simulink model "FIRST_SIMULATION"  (R2016a)
settings: Solver=ode45  SolverMode=SingleTasking  StartTime=0.0  StopTime=5/60  RelTol=1e-3
libraries: powerlib x63, powerlib_meascontrol x44
settings Model: Creator=hiago  LastModifiedBy=hiago
settings DebuggingCC: SFUnexpectedBacktrackingDiag=error  SFNoUnconditionalDefaultTransitionDiag=error
settings SFSimCC: SimUseLocalCustomCode=on
settings RTWCC: RTWUseLocalCustomCode=on
settings GRTTargetCC: TargetLangStandard=C99 (ISO)  GeneratePreprocessorConditionals=Use local settings
settings ConfigComp: CovMetricSettings=dwe  CovHtmlReporting=off  CovSaveCumulativeToWorkspaceVar=off  CovSaveSingleToWorkspaceVar=off  CovExternalEMLEnable=on

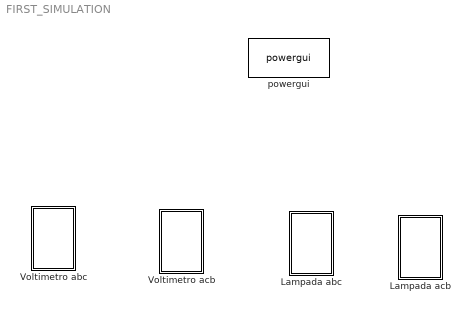
== system FIRST_SIMULATION ==
  Lampada abc : Subsystem
  Lampada acb : Subsystem
  Voltimetro abc : Subsystem
  Voltimetro acb : Subsystem
  powergui : powerlib/powergui  Priority=1  SimulationMode=Discrete  SampleTime=50e-6  frequency=60  Iterations=50  frequencyindice=60  Pbase=100e6  ErrMax=1e-4  UnitsV=kV  UnitsW=MW  buscounter=0  FunctionMessages=off  echomessages=off  EnableUseOfTLC=off  CurrentSourceSwitches=off  DisableSnubberDevices=off  DisableRonSwitches=off  DisableVfSwitches=off  DisplayEquations=off  SolverType=Tustin/Backward Euler (TBE)  Interpol=off  ExternalGateDelay=off  methode=off  Ts=100  x0status=blocks  SPID=on  SwTol=0  HookPort=off  RestoreLinks=warning  ResistiveCurrentMeasurement=off  Frange=[0:2:500]  Ylog=off  Xlog=on  ShowGrid=off  save=off  variable=ZData  structure=0  ZoomFFT=off  StartTime=0.0  cycles=1  DisplayStyle=1  fundamental=60  FreqAxis=off  MaxFrequency=1000  frequencyindicesteady=1  RmsSteady=1  display=off

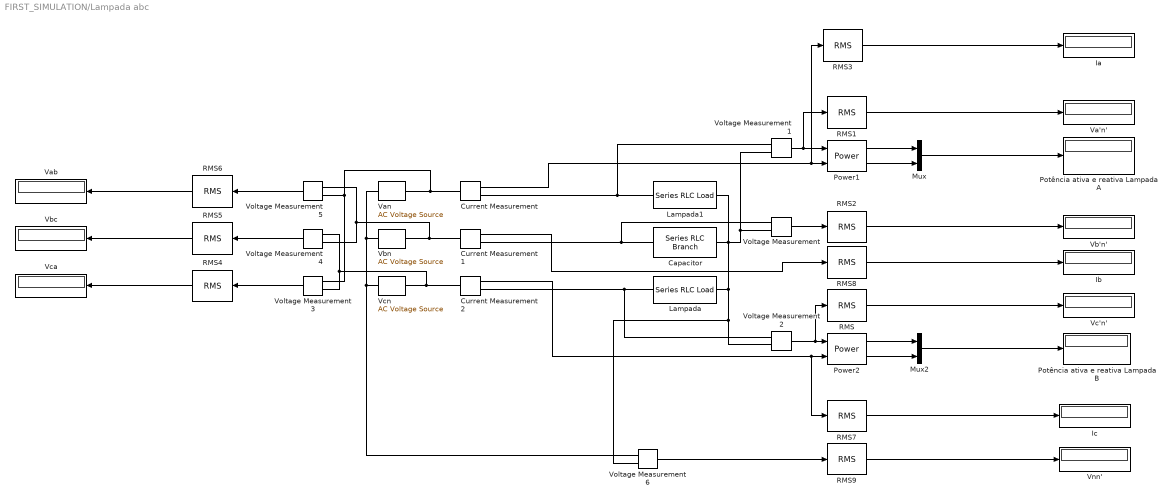
== system FIRST_SIMULATION/Lampada abc ==
  Capacitor : powerlib/Elements/Series RLC Branch  LConnTagsString=__new0  RConnTagsString=__new0  BranchType=RC  Resistance=0.0000001  Inductance=1e-3  SetiL0=off  InitialCurrent=0  Capacitance=25e-6  Setx0=off  InitialVoltage=0  Measurements=None
  Current Measurement : powerlib/Measurements/Current Measurement  PhasorSimulation=off  OutputType=Complex  PSBequivalent=0
  Current Measurement1 : powerlib/Measurements/Current Measurement  PhasorSimulation=off  OutputType=Complex  PSBequivalent=0
  Current Measurement2 : powerlib/Measurements/Current Measurement  PhasorSimulation=off  OutputType=Complex  PSBequivalent=0
  Ia : Display
  Ib : Display
  Ic : Display
  Lampada : powerlib/Elements/Series RLC Load  LConnTagsString=a  RConnTagsString=__new0  NominalVoltage=220  NominalFrequency=60  ActivePower=150  InductivePower=0  CapacitivePower=0  Setx0=off  InitialVoltage=0  SetiL0=off  InitialCurrent=0  Measurements=None  LoadType=constant Z
  Lampada1 : powerlib/Elements/Series RLC Load  LConnTagsString=a  RConnTagsString=__new0  NominalVoltage=220  NominalFrequency=60  ActivePower=150  InductivePower=0  CapacitivePower=0  Setx0=off  InitialVoltage=0  SetiL0=off  InitialCurrent=0  Measurements=None  LoadType=constant Z
  Mux : Mux  Inputs=2
  Mux2 : Mux  Inputs=2
  Potência ativa e reativa Lampada A : Display
  Potência ativa e reativa Lampada B : Display
  Power1 : powerlib_meascontrol/Measurements/Power  Freq=60  Vinit=[1, 0]  Iinit=[1, 0]  Ts=5e-5
  Power2 : powerlib_meascontrol/Measurements/Power  Freq=60  Vinit=[1, 0]  Iinit=[1, 0]  Ts=5e-5
  RMS{,1..9} (10 alike) : powerlib_meascontrol/Measurements/RMS  TrueRMS=on  Freq=60  RMSInit=120  Ts=5e-5
  Va'n' : Display
  Vab : Display
  Van : powerlib/Electrical Sources/AC Voltage Source  Amplitude=127*sqrt(2)  Phase=0  Frequency=60  SampleTime=5e-5  Measurements=None  BusType=swing  Pref=10e3  Qref=0  Qmin=-inf  Qmax=+inf
  Vb'n' : Display
  Vbc : Display
  Vbn : powerlib/Electrical Sources/AC Voltage Source  Amplitude=127*sqrt(2)  Phase=-120  Frequency=60  SampleTime=5e-5  Measurements=None  BusType=swing  Pref=10e3  Qref=0  Qmin=-inf  Qmax=+inf
  Vc'n' : Display
  Vca : Display
  Vcn : powerlib/Electrical Sources/AC Voltage Source  Amplitude=127*sqrt(2)  Phase=120  Frequency=60  SampleTime=5e-5  Measurements=None  BusType=swing  Pref=10e3  Qref=0  Qmin=-inf  Qmax=+inf
  Vnn' : Display
  Voltage Measurement{,1..6} (7 alike) : powerlib/Measurements/Voltage Measurement  PhasorSimulation=off  OutputType=Complex  PSBequivalent=0
  wires:
  Voltage Measurement2/1 -> RMS/1, Power2/1
  Current Measurement2/1 -> RMS7/1, Power2/2
  Voltage Measurement1/1 -> RMS1/1, Power1/1
  Current Measurement/1 -> RMS3/1, Power1/2
  Voltage Measurement/1 -> RMS2/1
  RMS1/1 -> Va'n'/1
  RMS2/1 -> Vb'n'/1
  RMS/1 -> Vc'n'/1
  Power1/1 -> Mux/1
  Power1/2 -> Mux/2
  Power2/1 -> Mux2/1
  Power2/2 -> Mux2/2
  Mux2/1 -> Potência ativa e reativa Lampada B/1
  Mux/1 -> Potência ativa e reativa Lampada A/1
  RMS6/1 -> Vab/1
  RMS5/1 -> Vbc/1
  Voltage Measurement3/1 -> RMS4/1
  Voltage Measurement5/1 -> RMS6/1
  Voltage Measurement4/1 -> RMS5/1
  RMS4/1 -> Vca/1
  RMS3/1 -> Ia/1
  RMS7/1 -> Ic/1
  RMS8/1 -> Ib/1
  Current Measurement1/1 -> RMS8/1
  RMS9/1 -> Vnn'/1
  Voltage Measurement6/1 -> RMS9/1
  connections:
  Lampada/LConn1 -- Current Measurement2/RConn1 -- Voltage Measurement2/LConn1
  Lampada1/RConn1 -- Voltage Measurement6/LConn2 -- Voltage Measurement2/LConn2 -- Lampada/RConn1 -- Voltage Measurement/LConn2 -- Voltage Measurement1/LConn2 -- Capacitor/RConn1
  Vcn/LConn1 -- Voltage Measurement6/LConn1 -- Van/LConn1 -- Vbn/LConn1
  Current Measurement/LConn1 -- Voltage Measurement3/LConn2 -- Voltage Measurement5/LConn1 -- Van/RConn1
  Current Measurement/RConn1 -- Voltage Measurement1/LConn1 -- Lampada1/LConn1
  Current Measurement1/LConn1 -- Voltage Measurement4/LConn1 -- Voltage Measurement5/LConn2 -- Vbn/RConn1
  Current Measurement1/RConn1 -- Voltage Measurement/LConn1 -- Capacitor/LConn1
  Current Measurement2/LConn1 -- Voltage Measurement3/LConn1 -- Voltage Measurement4/LConn2 -- Vcn/RConn1

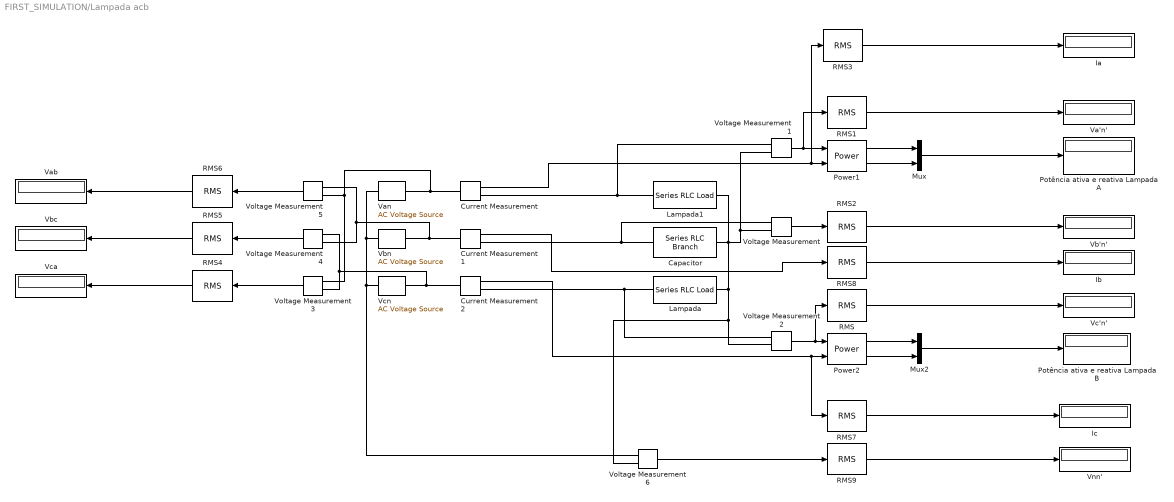
== system FIRST_SIMULATION/Lampada acb ==
  Capacitor : powerlib/Elements/Series RLC Branch  LConnTagsString=__new0  RConnTagsString=__new0  BranchType=RC  Resistance=0.0000001  Inductance=1e-3  SetiL0=off  InitialCurrent=0  Capacitance=25e-6  Setx0=off  InitialVoltage=0  Measurements=None
  Current Measurement : powerlib/Measurements/Current Measurement  PhasorSimulation=off  OutputType=Complex  PSBequivalent=0
  Current Measurement1 : powerlib/Measurements/Current Measurement  PhasorSimulation=off  OutputType=Complex  PSBequivalent=0
  Current Measurement2 : powerlib/Measurements/Current Measurement  PhasorSimulation=off  OutputType=Complex  PSBequivalent=0
  Ia : Display
  Ib : Display
  Ic : Display
  Lampada : powerlib/Elements/Series RLC Load  LConnTagsString=a  RConnTagsString=__new0  NominalVoltage=220  NominalFrequency=60  ActivePower=150  InductivePower=0  CapacitivePower=0  Setx0=off  InitialVoltage=0  SetiL0=off  InitialCurrent=0  Measurements=None  LoadType=constant Z
  Lampada1 : powerlib/Elements/Series RLC Load  LConnTagsString=a  RConnTagsString=__new0  NominalVoltage=220  NominalFrequency=60  ActivePower=150  InductivePower=0  CapacitivePower=0  Setx0=off  InitialVoltage=0  SetiL0=off  InitialCurrent=0  Measurements=None  LoadType=constant Z
  Mux : Mux  Inputs=2
  Mux2 : Mux  Inputs=2
  Potência ativa e reativa Lampada A : Display
  Potência ativa e reativa Lampada B : Display
  Power1 : powerlib_meascontrol/Measurements/Power  Freq=60  Vinit=[1, 0]  Iinit=[1, 0]  Ts=5e-5
  Power2 : powerlib_meascontrol/Measurements/Power  Freq=60  Vinit=[1, 0]  Iinit=[1, 0]  Ts=5e-5
  RMS{,1..9} (10 alike) : powerlib_meascontrol/Measurements/RMS  TrueRMS=on  Freq=60  RMSInit=120  Ts=5e-5
  Va'n' : Display
  Vab : Display
  Van : powerlib/Electrical Sources/AC Voltage Source  Amplitude=127*sqrt(2)  Phase=0  Frequency=60  SampleTime=5e-5  Measurements=None  BusType=swing  Pref=10e3  Qref=0  Qmin=-inf  Qmax=+inf
  Vb'n' : Display
  Vbc : Display
  Vbn : powerlib/Electrical Sources/AC Voltage Source  Amplitude=127*sqrt(2)  Phase=120  Frequency=60  SampleTime=5e-5  Measurements=None  BusType=swing  Pref=10e3  Qref=0  Qmin=-inf  Qmax=+inf
  Vc'n' : Display
  Vca : Display
  Vcn : powerlib/Electrical Sources/AC Voltage Source  Amplitude=127*sqrt(2)  Phase=-120  Frequency=60  SampleTime=5e-5  Measurements=None  BusType=swing  Pref=10e3  Qref=0  Qmin=-inf  Qmax=+inf
  Vnn' : Display
  Voltage Measurement{,1..6} (7 alike) : powerlib/Measurements/Voltage Measurement  PhasorSimulation=off  OutputType=Complex  PSBequivalent=0
  wires:
  RMS3/1 -> Ia/1
  Voltage Measurement2/1 -> RMS/1, Power2/1
  Voltage Measurement1/1 -> RMS1/1, Power1/1
  Current Measurement1/1 -> RMS8/1
  Power1/1 -> Mux/1
  RMS2/1 -> Vb'n'/1
  RMS6/1 -> Vab/1
  RMS4/1 -> Vca/1
  Power1/2 -> Mux/2
  Mux/1 -> Potência ativa e reativa Lampada A/1
  RMS9/1 -> Vnn'/1
  Voltage Measurement4/1 -> RMS5/1
  RMS8/1 -> Ib/1
  Voltage Measurement6/1 -> RMS9/1
  RMS1/1 -> Va'n'/1
  Voltage Measurement5/1 -> RMS6/1
  Power2/1 -> Mux2/1
  Mux2/1 -> Potência ativa e reativa Lampada B/1
  Voltage Measurement/1 -> RMS2/1
  RMS/1 -> Vc'n'/1
  RMS5/1 -> Vbc/1
  Voltage Measurement3/1 -> RMS4/1
  Power2/2 -> Mux2/2
  Current Measurement2/1 -> RMS7/1, Power2/2
  Current Measurement/1 -> RMS3/1, Power1/2
  RMS7/1 -> Ic/1
  connections:
  Voltage Measurement1/LConn2 -- Voltage Measurement/LConn2 -- Voltage Measurement6/LConn2 -- Voltage Measurement2/LConn2 -- Lampada/RConn1 -- Lampada1/RConn1 -- Capacitor/RConn1
  Voltage Measurement2/LConn1 -- Lampada/LConn1 -- Current Measurement2/RConn1
  Current Measurement/LConn1 -- Voltage Measurement3/LConn2 -- Voltage Measurement5/LConn1 -- Van/RConn1
  Vcn/LConn1 -- Voltage Measurement6/LConn1 -- Van/LConn1 -- Vbn/LConn1
  Current Measurement/RConn1 -- Voltage Measurement1/LConn1 -- Lampada1/LConn1
  Current Measurement1/RConn1 -- Voltage Measurement/LConn1 -- Capacitor/LConn1
  Current Measurement1/LConn1 -- Voltage Measurement4/LConn1 -- Voltage Measurement5/LConn2 -- Vbn/RConn1
  Current Measurement2/LConn1 -- Voltage Measurement3/LConn1 -- Voltage Measurement4/LConn2 -- Vcn/RConn1

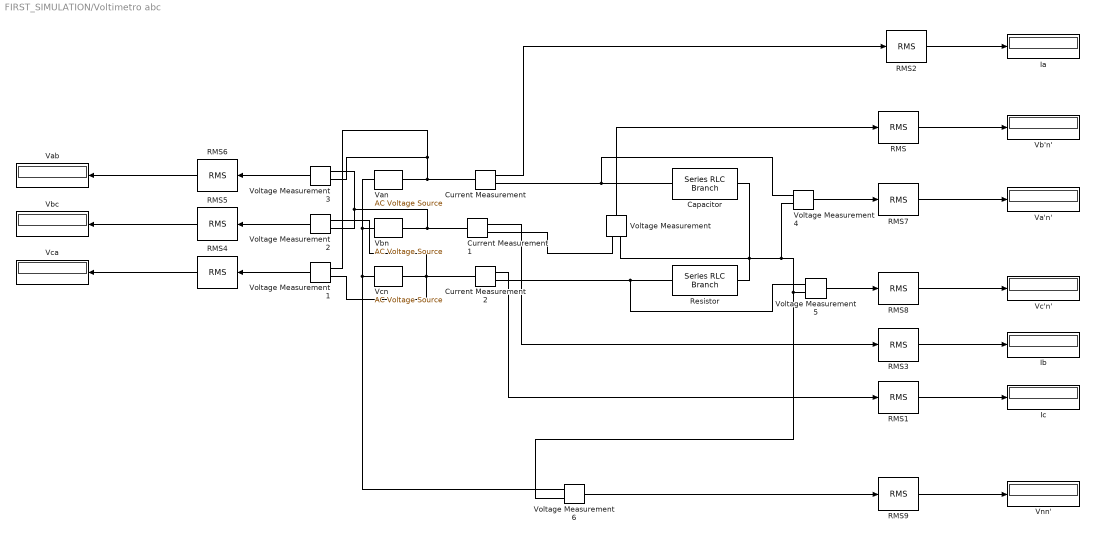
== system FIRST_SIMULATION/Voltimetro abc ==
  Capacitor : powerlib/Elements/Series RLC Branch  LConnTagsString=__new0  RConnTagsString=__new0  BranchType=RC  Resistance=0.0000001  Inductance=1e-3  SetiL0=off  InitialCurrent=0  Capacitance=25e-6  Setx0=off  InitialVoltage=0  Measurements=None
  Current Measurement : powerlib/Measurements/Current Measurement  PhasorSimulation=off  OutputType=Complex  PSBequivalent=0
  Current Measurement1 : powerlib/Measurements/Current Measurement  PhasorSimulation=off  OutputType=Complex  PSBequivalent=0
  Current Measurement2 : powerlib/Measurements/Current Measurement  PhasorSimulation=off  OutputType=Complex  PSBequivalent=0
  Ia : Display
  Ib : Display
  Ic : Display
  RMS{,1..9} (10 alike) : powerlib_meascontrol/Measurements/RMS  TrueRMS=on  Freq=60  RMSInit=120  Ts=5e-5
  Resistor : powerlib/Elements/Series RLC Branch  LConnTagsString=__new0  RConnTagsString=__new0  BranchType=R  Resistance=100  Inductance=1e-3  SetiL0=off  InitialCurrent=0  Capacitance=1e-6  Setx0=off  InitialVoltage=0  Measurements=None
  Va'n' : Display
  Vab : Display
  Van : powerlib/Electrical Sources/AC Voltage Source  Amplitude=127*sqrt(2)  Phase=0  Frequency=60  SampleTime=5e-5  Measurements=None  BusType=swing  Pref=10e3  Qref=0  Qmin=-inf  Qmax=+inf
  Vb'n' : Display
  Vbc : Display
  Vbn : powerlib/Electrical Sources/AC Voltage Source  Amplitude=127*sqrt(2)  Phase=-120  Frequency=60  SampleTime=5e-5  Measurements=None  BusType=swing  Pref=10e3  Qref=0  Qmin=-inf  Qmax=+inf
  Vc'n' : Display
  Vca : Display
  Vcn : powerlib/Electrical Sources/AC Voltage Source  Amplitude=127*sqrt(2)  Phase=120  Frequency=60  SampleTime=5e-5  Measurements=None  BusType=swing  Pref=10e3  Qref=0  Qmin=-inf  Qmax=+inf
  Vnn' : Display
  Voltage Measurement{,1..6} (7 alike) : powerlib/Measurements/Voltage Measurement  PhasorSimulation=off  OutputType=Complex  PSBequivalent=0
  wires:
  Voltage Measurement3/1 -> RMS6/1
  RMS8/1 -> Vc'n'/1
  RMS4/1 -> Vca/1
  Voltage Measurement6/1 -> RMS9/1
  RMS9/1 -> Vnn'/1
  RMS1/1 -> Ic/1
  Voltage Measurement5/1 -> RMS8/1
  RMS2/1 -> Ia/1
  RMS/1 -> Vb'n'/1
  Voltage Measurement2/1 -> RMS5/1
  RMS5/1 -> Vbc/1
  RMS6/1 -> Vab/1
  RMS3/1 -> Ib/1
  RMS7/1 -> Va'n'/1
  Current Measurement1/1 -> RMS3/1
  Voltage Measurement1/1 -> RMS4/1
  Voltage Measurement/1 -> RMS/1
  Current Measurement/1 -> RMS2/1
  Voltage Measurement4/1 -> RMS7/1
  Current Measurement2/1 -> RMS1/1
  connections:
  Current Measurement/RConn1 -- Voltage Measurement4/LConn1 -- Capacitor/LConn1
  Current Measurement/LConn1 -- Van/RConn1 -- Voltage Measurement3/LConn1 -- Voltage Measurement1/LConn2
  Current Measurement2/RConn1 -- Voltage Measurement5/LConn1 -- Resistor/LConn1
  Vbn/LConn1 -- Van/LConn1 -- Voltage Measurement6/LConn1 -- Vcn/LConn1
  Voltage Measurement3/LConn2 -- Voltage Measurement2/LConn1 -- Vbn/RConn1 -- Current Measurement1/LConn1
  Voltage Measurement/LConn2 -- Voltage Measurement5/LConn2 -- Voltage Measurement6/LConn2 -- Voltage Measurement4/LConn2 -- Resistor/RConn1 -- Capacitor/RConn1
  Current Measurement2/LConn1 -- Voltage Measurement2/LConn2 -- Voltage Measurement1/LConn1 -- Vcn/RConn1
  Current Measurement1/RConn1 -- Voltage Measurement/LConn1

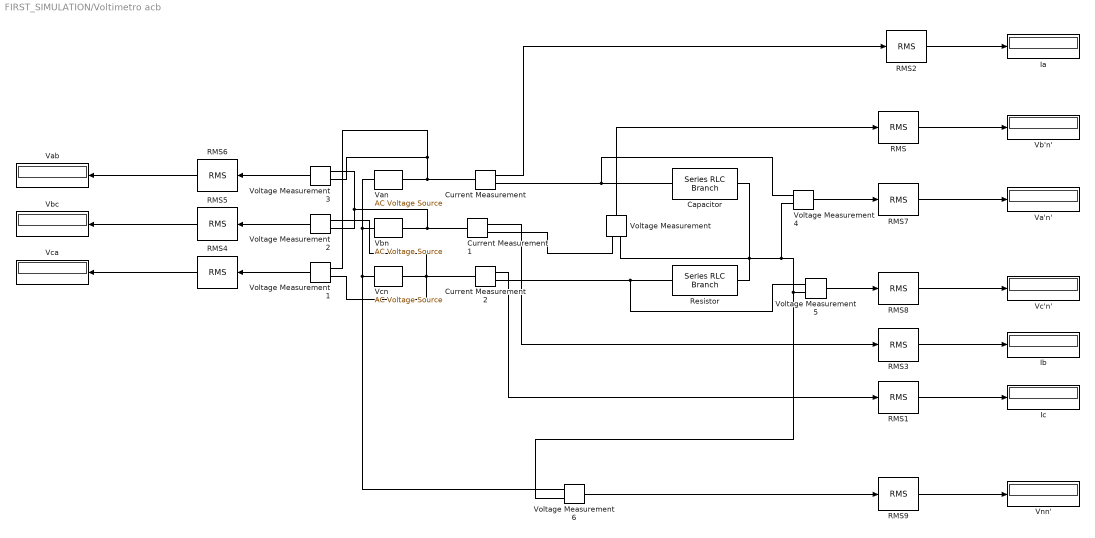
== system FIRST_SIMULATION/Voltimetro acb ==
  Capacitor : powerlib/Elements/Series RLC Branch  LConnTagsString=__new0  RConnTagsString=__new0  BranchType=RC  Resistance=0.0000001  Inductance=1e-3  SetiL0=off  InitialCurrent=0  Capacitance=25e-6  Setx0=off  InitialVoltage=0  Measurements=None
  Current Measurement : powerlib/Measurements/Current Measurement  PhasorSimulation=off  OutputType=Complex  PSBequivalent=0
  Current Measurement1 : powerlib/Measurements/Current Measurement  PhasorSimulation=off  OutputType=Complex  PSBequivalent=0
  Current Measurement2 : powerlib/Measurements/Current Measurement  PhasorSimulation=off  OutputType=Complex  PSBequivalent=0
  Ia : Display
  Ib : Display
  Ic : Display
  RMS{,1..9} (10 alike) : powerlib_meascontrol/Measurements/RMS  TrueRMS=on  Freq=60  RMSInit=120  Ts=5e-5
  Resistor : powerlib/Elements/Series RLC Branch  LConnTagsString=__new0  RConnTagsString=__new0  BranchType=R  Resistance=100  Inductance=1e-3  SetiL0=off  InitialCurrent=0  Capacitance=1e-6  Setx0=off  InitialVoltage=0  Measurements=None
  Va'n' : Display
  Vab : Display
  Van : powerlib/Electrical Sources/AC Voltage Source  Amplitude=127*sqrt(2)  Phase=0  Frequency=60  SampleTime=5e-5  Measurements=None  BusType=swing  Pref=10e3  Qref=0  Qmin=-inf  Qmax=+inf
  Vb'n' : Display
  Vbc : Display
  Vbn : powerlib/Electrical Sources/AC Voltage Source  Amplitude=127*sqrt(2)  Phase=120  Frequency=60  SampleTime=5e-5  Measurements=None  BusType=swing  Pref=10e3  Qref=0  Qmin=-inf  Qmax=+inf
  Vc'n' : Display
  Vca : Display
  Vcn : powerlib/Electrical Sources/AC Voltage Source  Amplitude=127*sqrt(2)  Phase=-120  Frequency=60  SampleTime=5e-5  Measurements=None  BusType=swing  Pref=10e3  Qref=0  Qmin=-inf  Qmax=+inf
  Vnn' : Display
  Voltage Measurement{,1..6} (7 alike) : powerlib/Measurements/Voltage Measurement  PhasorSimulation=off  OutputType=Complex  PSBequivalent=0
  wires:
  Voltage Measurement2/1 -> RMS5/1
  Voltage Measurement5/1 -> RMS8/1
  RMS6/1 -> Vab/1
  Current Measurement2/1 -> RMS1/1
  Current Measurement1/1 -> RMS3/1
  Voltage Measurement/1 -> RMS/1
  Voltage Measurement1/1 -> RMS4/1
  RMS2/1 -> Ia/1
  RMS3/1 -> Ib/1
  Voltage Measurement6/1 -> RMS9/1
  RMS9/1 -> Vnn'/1
  Current Measurement/1 -> RMS2/1
  RMS5/1 -> Vbc/1
  RMS/1 -> Vb'n'/1
  RMS8/1 -> Vc'n'/1
  RMS1/1 -> Ic/1
  Voltage Measurement3/1 -> RMS6/1
  Voltage Measurement4/1 -> RMS7/1
  RMS4/1 -> Vca/1
  RMS7/1 -> Va'n'/1
  connections:
  Voltage Measurement/LConn2 -- Voltage Measurement5/LConn2 -- Voltage Measurement6/LConn2 -- Voltage Measurement4/LConn2 -- Resistor/RConn1 -- Capacitor/RConn1
  Voltage Measurement3/LConn2 -- Voltage Measurement2/LConn1 -- Vbn/RConn1 -- Current Measurement1/LConn1
  Current Measurement2/LConn1 -- Voltage Measurement2/LConn2 -- Voltage Measurement1/LConn1 -- Vcn/RConn1
  Vbn/LConn1 -- Voltage Measurement6/LConn1 -- Vcn/LConn1 -- Van/LConn1
  Current Measurement/LConn1 -- Voltage Measurement3/LConn1 -- Voltage Measurement1/LConn2 -- Van/RConn1
  Current Measurement2/RConn1 -- Voltage Measurement5/LConn1 -- Resistor/LConn1
  Current Measurement/RConn1 -- Voltage Measurement4/LConn1 -- Capacitor/LConn1
  Current Measurement1/RConn1 -- Voltage Measurement/LConn1
